simulink model "SOH_OL_Harness"  (R2024b)
settings: Solver=FixedStepAuto  StartTime=0.0  StopTime=sim_time  FixedStep=sample_time  RelTol=1e-3  EnableMultiTasking=on
libraries: simulink x1
settings Model: Creator=favv5g  LastModifiedBy=voillat
settings SolverCC: AlgebraicLoopSolver=TrustRegion
settings DataIOCC: LimitDataPoints=on
settings OptimizationCC: LifeSpan=inf
settings DebuggingCC: UnconnectedInputMsg=warning  UnconnectedOutputMsg=warning  UnconnectedLineMsg=warning  AllowSymbolicDim=off  SFUnexpectedBacktrackingDiag=warning  SFNoUnconditionalDefaultTransitionDiag=warning  SFExecutionAtInitializationDiag=none  ArithmeticOperatorsInVariantConditions=warning
settings ModelReferenceCC: EnableRefExpFcnMdlSchedulingChecks=on  PropagateSignalLabelsOutOfModel=off
settings SFSimCC: SimUseLocalCustomCode=off  CustomCodeUndefinedFunction=UseInterfaceOnly
settings RTWCC: RTWUseLocalCustomCode=off  GPUComputeCapability=3.5
settings CodeAppCC: StateflowObjectComments=on
settings GRTTargetCC: TargetLangStandard=C89/C90 (ANSI)
settings ConfigComp: CovMetricSettings=dw  CovSaveCumulativeToWorkspaceVar=on  CovSaveSingleToWorkspaceVar=on  CovExternalEMLEnable=off

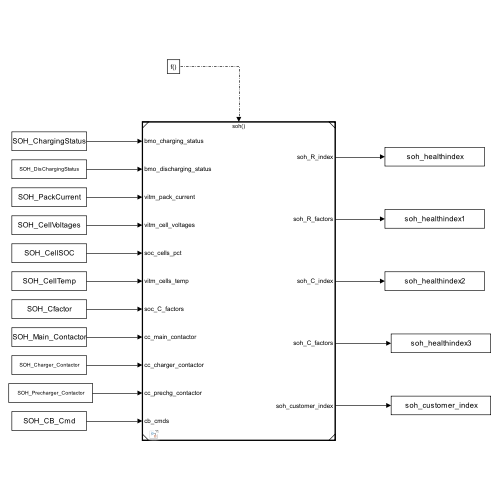
[thumbnail: Simulink's stored preview of the top-level diagram]
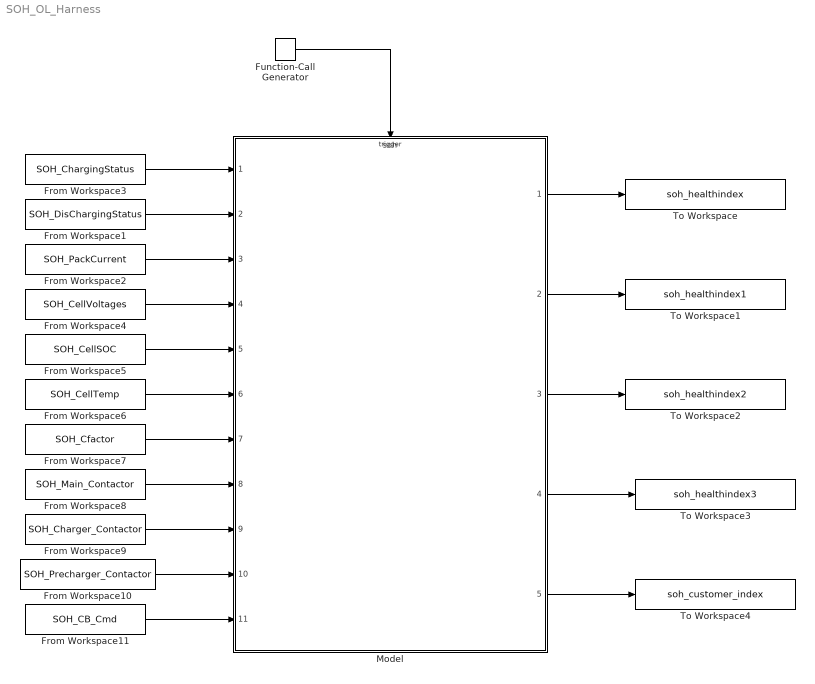
== system SOH_OL_Harness ==
  From Workspace1 : FromWorkspace  VariableName=SOH_DisChargingStatus  SampleTime=-1
  From Workspace10 : FromWorkspace  VariableName=SOH_Precharger_Contactor  SampleTime=-1
  From Workspace11 : FromWorkspace  VariableName=SOH_CB_Cmd  SampleTime=-1
  From Workspace2 : FromWorkspace  VariableName=SOH_PackCurrent  SampleTime=-1
  From Workspace3 : FromWorkspace  VariableName=SOH_ChargingStatus  SampleTime=-1
  From Workspace4 : FromWorkspace  VariableName=SOH_CellVoltages  SampleTime=-1
  From Workspace5 : FromWorkspace  VariableName=SOH_CellSOC  SampleTime=-1
  From Workspace6 : FromWorkspace  VariableName=SOH_CellTemp  SampleTime=-1
  From Workspace7 : FromWorkspace  VariableName=SOH_Cfactor  SampleTime=-1
  From Workspace8 : FromWorkspace  VariableName=SOH_Main_Contactor  SampleTime=-1
  From Workspace9 : FromWorkspace  VariableName=SOH_Charger_Contactor  SampleTime=-1
  Function-Call Generator : simulink/Ports & Subsystems/Function-Call Generator  sample_time=0.01  numberOfIterations=1  DisallowWideOutput=off
  Model : ModelReference  ModelNameDialog=soh.slx  SimulationMode=Normal  ModelReferenceVersion=15.2  TriggerPortName=Trigger  TriggerPortTriggerType=function-call  TriggerPortStatesWhenEnabling=held
  To Workspace : ToWorkspace  VariableName=soh_healthindex  SaveFormat=Timeseries  SampleTime=-1
  To Workspace1 : ToWorkspace  VariableName=soh_healthindex1  SaveFormat=Timeseries  SampleTime=-1
  To Workspace2 : ToWorkspace  VariableName=soh_healthindex2  SaveFormat=Timeseries  SampleTime=-1
  To Workspace3 : ToWorkspace  VariableName=soh_healthindex3  SaveFormat=Timeseries  SampleTime=-1
  To Workspace4 : ToWorkspace  VariableName=soh_customer_index  SaveFormat=Timeseries  SampleTime=-1
  wires:
  From Workspace3/1 -> Model/1
  From Workspace1/1 -> Model/2
  From Workspace2/1 -> Model/3
  From Workspace4/1 -> Model/4
  From Workspace5/1 -> Model/5
  From Workspace6/1 -> Model/6
  Model/1 -> To Workspace/1
  Function-Call Generator/1 -> Model/Trigger
  From Workspace7/1 -> Model/7
  Model/2 -> To Workspace1/1
  Model/3 -> To Workspace2/1
  Model/4 -> To Workspace3/1
  From Workspace8/1 -> Model/8
  From Workspace9/1 -> Model/9
  From Workspace10/1 -> Model/10
  From Workspace11/1 -> Model/11
  Model/5 -> To Workspace4/1
